simulink model "firefliesDemo"  (Simulink 7.4)
settings: Solver=ode3  StartTime=0.0  StopTime=200  FixedStep=1  RelTol=1e-3
values from neighbouring files (symbols this model uses):
  K = 2.5    [firefliesDemo.mat]
  N = 5    [clusterDemo.mat]    (also in firefliesDemo.mat = 10)
  omega = 0.628318530718    [firefliesDemo.mat]
  rho0 = 10    [firefliesDemo.mat]
  threshold = 0.8    [firefliesDemo.mat]
  var = 0    [clusterDemo.mat]    (also in firefliesDemo.mat = 3)
(part 1 of 2)
settings Model: Creator=chepeadan  LastModifiedBy=chepeadan

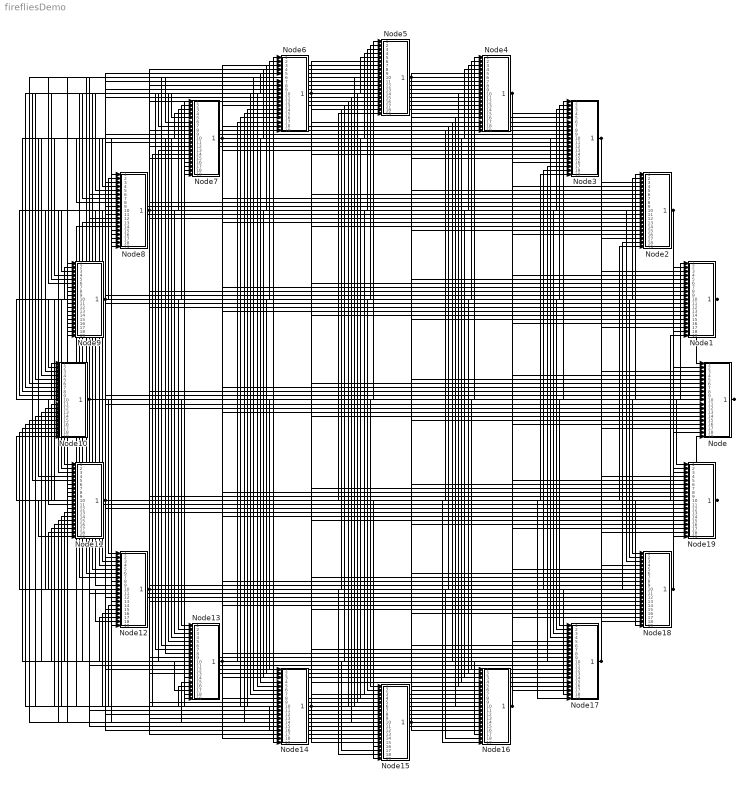
== system firefliesDemo ==
  Node : Subsystem
  Node1 : Subsystem
  Node10 : Subsystem
  Node11 : Subsystem
  Node12 : Subsystem
  Node13 : Subsystem
  Node14 : Subsystem
  Node15 : Subsystem
  Node16 : Subsystem
  Node17 : Subsystem
  Node18 : Subsystem
  Node19 : Subsystem
  Node2 : Subsystem
  Node3 : Subsystem
  Node4 : Subsystem
  Node5 : Subsystem
  Node6 : Subsystem
  Node7 : Subsystem
  Node8 : Subsystem
  Node9 : Subsystem
  wires:
  Node/1(Out1) -> Node1/1(In1), Node2/1(In1), Node3/1(In1), Node4/1(In1), Node5/1(In1), Node6/1(In1), Node7/1(In1), Node8/1(In1), Node9/1(In1), Node10/1(In1), Node11/1(In1), Node12/1(In1), Node13/1(In1), Node14/1(In1), Node15/1(In1), Node16/1(In1), Node17/1(In1), Node18/1(In1), Node19/1(In1)
  Node1/1(Out1) -> Node/1(In2), Node2/2(In2), Node3/2(In2), Node4/2(In2), Node5/2(In2), Node6/2(In2), Node7/2(In2), Node8/2(In2), Node9/2(In2), Node10/2(In2), Node11/2(In2), Node12/2(In2), Node13/2(In2), Node14/2(In2), Node15/2(In2), Node16/2(In2), Node17/2(In2), Node18/2(In2), Node19/2(In2)
  Node2/1(Out1) -> Node/2(In3), Node1/2(In3), Node3/3(In3), Node4/3(In3), Node5/3(In3), Node6/3(In3), Node7/3(In3), Node8/3(In3), Node9/3(In3), Node10/3(In3), Node11/3(In3), Node12/3(In3), Node13/3(In3), Node14/3(In3), Node15/3(In3), Node16/3(In3), Node17/3(In3), Node18/3(In3), Node19/3(In3)
  Node3/1(Out1) -> Node/3(In4), Node1/3(In4), Node2/3(In4), Node4/4(In4), Node5/4(In4), Node6/4(In4), Node7/4(In4), Node8/4(In4), Node9/4(In4), Node10/4(In4), Node11/4(In4), Node12/4(In4), Node13/4(In4), Node14/4(In4), Node15/4(In4), Node16/4(In4), Node17/4(In4), Node18/4(In4), Node19/4(In4)
  Node4/1(Out1) -> Node/4(In5), Node1/4(In5), Node2/4(In5), Node3/4(In5), Node5/5(In5), Node6/5(In5), Node7/5(In5), Node8/5(In5), Node9/5(In5), Node10/5(In5), Node11/5(In5), Node12/5(In5), Node13/5(In5), Node14/5(In5), Node15/5(In5), Node16/5(In5), Node17/5(In5), Node18/5(In5), Node19/5(In5)
  Node5/1(Out1) -> Node/5(In6), Node1/5(In6), Node2/5(In6), Node3/5(In6), Node4/5(In6), Node6/6(In6), Node7/6(In6), Node8/6(In6), Node9/6(In6), Node10/6(In6), Node11/6(In6), Node12/6(In6), Node13/6(In6), Node14/6(In6), Node15/6(In6), Node16/6(In6), Node17/6(In6), Node18/6(In6), Node19/6(In6)
  Node6/1(Out1) -> Node/6(In7), Node1/6(In7), Node2/6(In7), Node3/6(In7), Node4/6(In7), Node5/6(In7), Node7/7(In7), Node8/7(In7), Node9/7(In7), Node10/7(In7), Node11/7(In7), Node12/7(In7), Node13/7(In7), Node14/7(In7), Node15/7(In7), Node16/7(In7), Node17/7(In7), Node18/7(In7), Node19/7(In7)
  Node7/1(Out1) -> Node/7(In8), Node1/7(In8), Node2/7(In8), Node3/7(In8), Node4/7(In8), Node5/7(In8), Node6/7(In8), Node8/8(In8), Node9/8(In8), Node10/8(In8), Node11/8(In8), Node12/8(In8), Node13/8(In8), Node14/8(In8), Node15/8(In8), Node16/8(In8), Node17/8(In8), Node18/8(In8), Node19/8(In8)
  Node8/1(Out1) -> Node/8(In9), Node1/8(In9), Node2/8(In9), Node3/8(In9), Node4/8(In9), Node5/8(In9), Node6/8(In9), Node7/8(In9), Node9/9(In9), Node10/9(In9), Node11/9(In9), Node12/9(In9), Node13/9(In9), Node14/9(In9), Node15/9(In9), Node16/9(In9), Node17/9(In9), Node18/9(In9), Node19/9(In9)
  Node9/1(Out1) -> Node/9(In10), Node1/9(In10), Node2/9(In10), Node3/9(In10), Node4/9(In10), Node5/9(In10), Node6/9(In10), Node7/9(In10), Node8/9(In10), Node10/10(In10), Node11/10(In10), Node12/10(In10), Node13/10(In10), Node14/10(In10), Node15/10(In10), Node16/10(In10), Node17/10(In10), Node18/10(In10), Node19/10(In10)
  Node10/1(Out1) -> Node/10(In11), Node1/10(In11), Node2/10(In11), Node3/10(In11), Node4/10(In11), Node5/10(In11), Node6/10(In11), Node7/10(In11), Node8/10(In11), Node9/10(In11), Node11/11(In11), Node12/11(In11), Node13/11(In11), Node14/11(In11), Node15/11(In11), Node16/11(In11), Node17/11(In11), Node18/11(In11), Node19/11(In11)
  Node11/1(Out1) -> Node/11(In12), Node1/11(In12), Node2/11(In12), Node3/11(In12), Node4/11(In12), Node5/11(In12), Node6/11(In12), Node7/11(In12), Node8/11(In12), Node9/11(In12), Node10/11(In12), Node12/12(In12), Node13/12(In12), Node14/12(In12), Node15/12(In12), Node16/12(In12), Node17/12(In12), Node18/12(In12), Node19/12(In12)
  Node12/1(Out1) -> Node/12(In13), Node1/12(In13), Node2/12(In13), Node3/12(In13), Node4/12(In13), Node5/12(In13), Node6/12(In13), Node7/12(In13), Node8/12(In13), Node9/12(In13), Node10/12(In13), Node11/12(In13), Node13/13(In13), Node14/13(In13), Node15/13(In13), Node16/13(In13), Node17/13(In13), Node18/13(In13), Node19/13(In13)
  Node13/1(Out1) -> Node/13(In14), Node1/13(In14), Node2/13(In14), Node3/13(In14), Node4/13(In14), Node5/13(In14), Node6/13(In14), Node7/13(In14), Node8/13(In14), Node9/13(In14), Node10/13(In14), Node11/13(In14), Node12/13(In14), Node14/14(In14), Node15/14(In14), Node16/14(In14), Node17/14(In14), Node18/14(In14), Node19/14(In14)
  Node14/1(Out1) -> Node/14(In15), Node1/14(In15), Node2/14(In15), Node3/14(In15), Node4/14(In15), Node5/14(In15), Node6/14(In15), Node7/14(In15), Node8/14(In15), Node9/14(In15), Node10/14(In15), Node11/14(In15), Node12/14(In15), Node13/14(In15), Node15/15(In15), Node16/15(In15), Node17/15(In15), Node18/15(In15), Node19/15(In15)
  Node15/1(Out1) -> Node/15(In16), Node1/15(In16), Node2/15(In16), Node3/15(In16), Node4/15(In16), Node5/15(In16), Node6/15(In16), Node7/15(In16), Node8/15(In16), Node9/15(In16), Node10/15(In16), Node11/15(In16), Node12/15(In16), Node13/15(In16), Node14/15(In16), Node16/16(In16), Node17/16(In16), Node18/16(In16), Node19/16(In16)
  Node16/1(Out1) -> Node/16(In17), Node1/16(In17), Node2/16(In17), Node3/16(In17), Node4/16(In17), Node5/16(In17), Node6/16(In17), Node7/16(In17), Node8/16(In17), Node9/16(In17), Node10/16(In17), Node11/16(In17), Node12/16(In17), Node13/16(In17), Node14/16(In17), Node15/16(In17), Node17/17(In17), Node18/17(In17), Node19/17(In17)
  Node17/1(Out1) -> Node/17(In18), Node1/17(In18), Node2/17(In18), Node3/17(In18), Node4/17(In18), Node5/17(In18), Node6/17(In18), Node7/17(In18), Node8/17(In18), Node9/17(In18), Node10/17(In18), Node11/17(In18), Node12/17(In18), Node13/17(In18), Node14/17(In18), Node15/17(In18), Node16/17(In18), Node18/18(In18), Node19/18(In18)
  Node18/1(Out1) -> Node/18(In19), Node1/18(In19), Node2/18(In19), Node3/18(In19), Node4/18(In19), Node5/18(In19), Node6/18(In19), Node7/18(In19), Node8/18(In19), Node9/18(In19), Node10/18(In19), Node11/18(In19), Node12/18(In19), Node13/18(In19), Node14/18(In19), Node15/18(In19), Node16/18(In19), Node17/18(In19), Node19/19(In19)
  Node19/1(Out1) -> Node/19(In20), Node1/19(In20), Node2/19(In20), Node3/19(In20), Node4/19(In20), Node5/19(In20), Node6/19(In20), Node7/19(In20), Node8/19(In20), Node9/19(In20), Node10/19(In20), Node11/19(In20), Node12/19(In20), Node13/19(In20), Node14/19(In20), Node15/19(In20), Node16/19(In20), Node17/19(In20), Node18/19(In20)

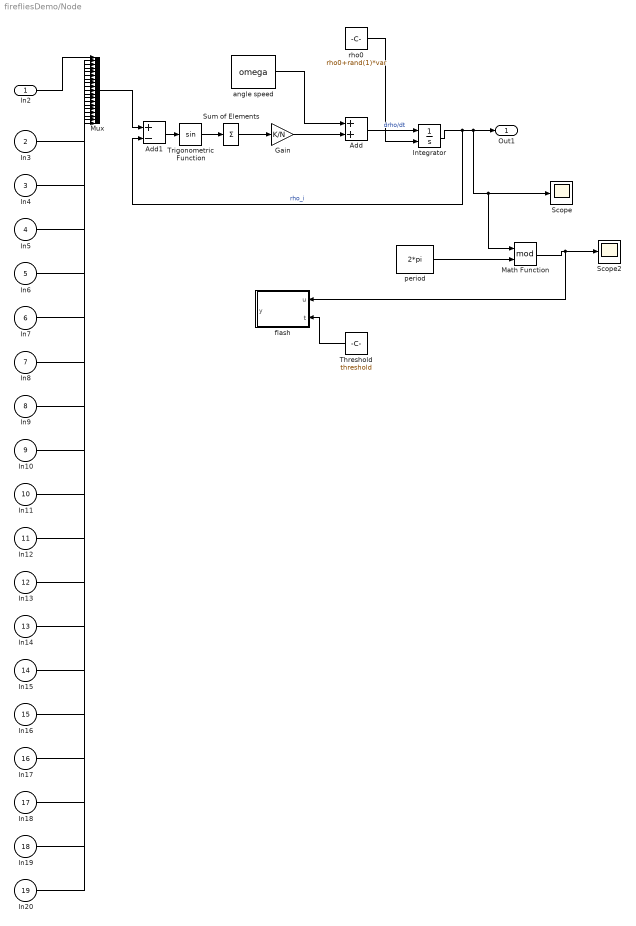
== system firefliesDemo/Node ==
  In2 : Inport  OutDataType=fixdt(1, 16)  OutScaling=2^0
  In3 : Inport  Port=2
  In4 : Inport  Port=3
  In5 : Inport  Port=4
  In6 : Inport  Port=5
  In7 : Inport  Port=6
  In8 : Inport  Port=7
  In9 : Inport  Port=8
  In10 : Inport  Port=9
  In11 : Inport  Port=10
  In12 : Inport  Port=11
  In13 : Inport  Port=12
  In14 : Inport  Port=13
  In15 : Inport  Port=14
  In16 : Inport  Port=15
  In17 : Inport  Port=16
  In18 : Inport  Port=17
  In19 : Inport  Port=18
  In20 : Inport  Port=19
  Add : Sum  OutDataType=fixdt(1, 16)  OutScaling=2^-10
  Add1 : Sum  Inputs=+-  OutDataType=fixdt(1, 16)  OutScaling=2^-10
  Gain : Gain  Gain=K/N  ParameterDataType=fixdt(1, 16)  ParameterScaling=2^0  OutDataType=fixdt(1, 16)  OutScaling=2^0
  Integrator : Integrator  InitialConditionSource=external
  Math Function : Math  Operator=mod  OutDataType=fixdt(1, 16)  OutScaling=2^0  SaturateOnIntegerOverflow=on
  Mux : Mux  Inputs=19
  Scope : Scope
  Scope2 : Scope
      settings: SaveName=ScopeData2
  Sum of Elements : Sum  Inputs=+  OutDataType=fixdt(1, 16)  OutScaling=2^-10
  Threshold : Constant  Value=threshold  OutDataType=fixdt(1, 16)  OutScaling=2^0
  Trigonometric Function : Trigonometry
  angle speed : Constant  Value=omega  OutDataType=fixdt(1, 16)  OutScaling=2^0
  flash : Stateflow chart
  period : Constant  Value=2*pi  OutDataType=fixdt(1, 16)  OutScaling=2^0
  rho0 : Constant  Value=rho0+rand(1)*var  OutDataType=fixdt(1, 16)  OutScaling=2^0
  Out1 : Outport  OutDataType=fixdt(1, 16)  OutScaling=2^0
  wires:
  In20/1 -> Mux/19
  In19/1 -> Mux/18
  In18/1 -> Mux/17
  In17/1 -> Mux/16
  In16/1 -> Mux/15
  In15/1 -> Mux/14
  In14/1 -> Mux/13
  In13/1 -> Mux/12
  In12/1 -> Mux/11
  In11/1 -> Mux/10
  In10/1 -> Mux/9
  In9/1 -> Mux/8
  In8/1 -> Mux/7
  In7/1 -> Mux/6
  In6/1 -> Mux/5
  In5/1 -> Mux/4
  In4/1 -> Mux/3
  In3/1 -> Mux/2
  Threshold/1 -> flash/2(t)
  Math Function/1 -> flash/1(u), Scope2/1
  period/1 -> Math Function/2
  rho0/1 -> Integrator/2
  Sum of Elements/1 -> Gain/1
  Trigonometric Function/1 -> Sum of Elements/1
  Add/1 -> Integrator/1  "drho/dt"
  Gain/1 -> Add/2
  angle speed/1 -> Add/1
  Add1/1 -> Trigonometric Function/1
  Integrator/1 -> Math Function/1, Scope/1, Out1/1, Add1/2  "rho_i"
  Mux/1 -> Add1/1
  In2/1 -> Mux/1

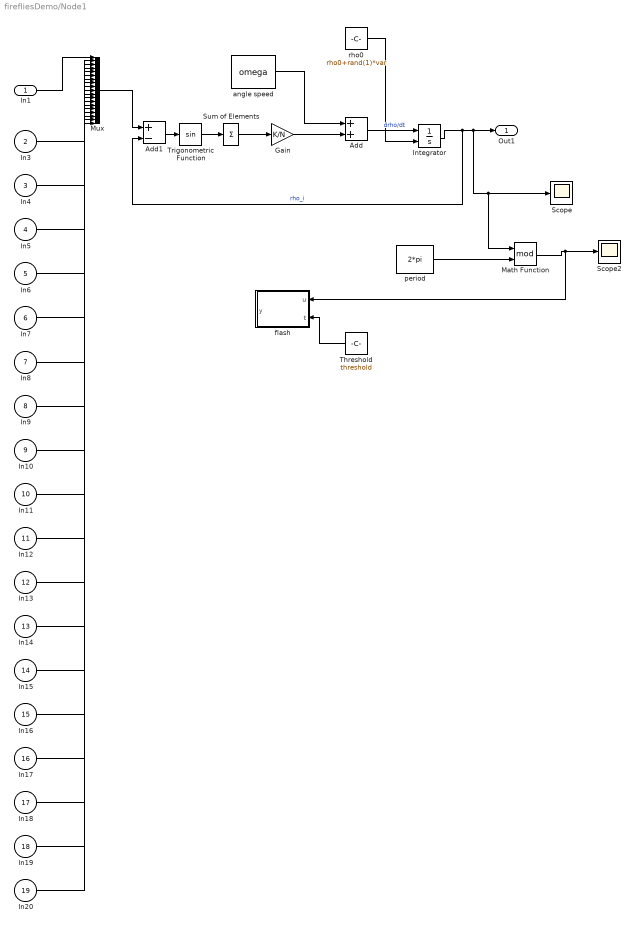
== system firefliesDemo/Node1 ==
  In1 : Inport  OutDataType=fixdt(1, 16)  OutScaling=2^0
  In3 : Inport  Port=2
  In4 : Inport  Port=3
  In5 : Inport  Port=4
  In6 : Inport  Port=5
  In7 : Inport  Port=6
  In8 : Inport  Port=7
  In9 : Inport  Port=8
  In10 : Inport  Port=9
  In11 : Inport  Port=10
  In12 : Inport  Port=11
  In13 : Inport  Port=12
  In14 : Inport  Port=13
  In15 : Inport  Port=14
  In16 : Inport  Port=15
  In17 : Inport  Port=16
  In18 : Inport  Port=17
  In19 : Inport  Port=18
  In20 : Inport  Port=19
  Add : Sum  OutDataType=fixdt(1, 16)  OutScaling=2^-10
  Add1 : Sum  Inputs=+-  OutDataType=fixdt(1, 16)  OutScaling=2^-10
  Gain : Gain  Gain=K/N  ParameterDataType=fixdt(1, 16)  ParameterScaling=2^0  OutDataType=fixdt(1, 16)  OutScaling=2^0
  Integrator : Integrator  InitialConditionSource=external
  Math Function : Math  Operator=mod  OutDataType=fixdt(1, 16)  OutScaling=2^0  SaturateOnIntegerOverflow=on
  Mux : Mux  Inputs=19
  Scope : Scope
  Scope2 : Scope
      settings: SaveName=ScopeData2
  Sum of Elements : Sum  Inputs=+  OutDataType=fixdt(1, 16)  OutScaling=2^-10
  Threshold : Constant  Value=threshold  OutDataType=fixdt(1, 16)  OutScaling=2^0
  Trigonometric Function : Trigonometry
  angle speed : Constant  Value=omega  OutDataType=fixdt(1, 16)  OutScaling=2^0
  flash : Stateflow chart
  period : Constant  Value=2*pi  OutDataType=fixdt(1, 16)  OutScaling=2^0
  rho0 : Constant  Value=rho0+rand(1)*var  OutDataType=fixdt(1, 16)  OutScaling=2^0
  Out1 : Outport  OutDataType=fixdt(1, 16)  OutScaling=2^0
  wires:
  In20/1 -> Mux/19
  In19/1 -> Mux/18
  In18/1 -> Mux/17
  In17/1 -> Mux/16
  In16/1 -> Mux/15
  In15/1 -> Mux/14
  In14/1 -> Mux/13
  In13/1 -> Mux/12
  In12/1 -> Mux/11
  In11/1 -> Mux/10
  In10/1 -> Mux/9
  In9/1 -> Mux/8
  In8/1 -> Mux/7
  In7/1 -> Mux/6
  In6/1 -> Mux/5
  In5/1 -> Mux/4
  In4/1 -> Mux/3
  In3/1 -> Mux/2
  Threshold/1 -> flash/2(t)
  Math Function/1 -> flash/1(u), Scope2/1
  period/1 -> Math Function/2
  rho0/1 -> Integrator/2
  Sum of Elements/1 -> Gain/1
  Trigonometric Function/1 -> Sum of Elements/1
  Add/1 -> Integrator/1  "drho/dt"
  Gain/1 -> Add/2
  angle speed/1 -> Add/1
  Add1/1 -> Trigonometric Function/1
  Integrator/1 -> Math Function/1, Scope/1, Out1/1, Add1/2  "rho_i"
  Mux/1 -> Add1/1
  In1/1 -> Mux/1

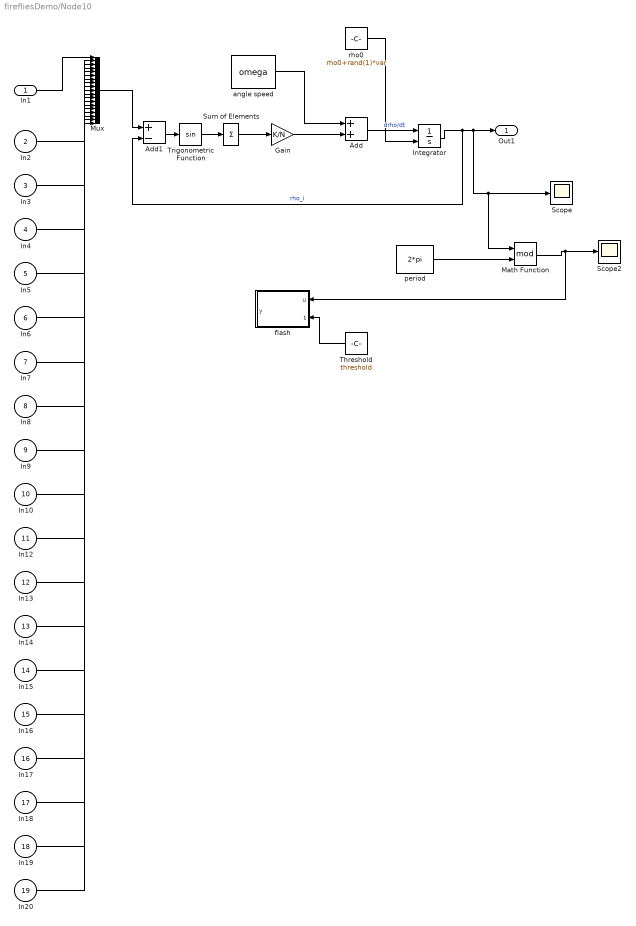
== system firefliesDemo/Node10 ==
  In1 : Inport  OutDataType=fixdt(1, 16)  OutScaling=2^0
  In2 : Inport  Port=2
  In3 : Inport  Port=3
  In4 : Inport  Port=4
  In5 : Inport  Port=5
  In6 : Inport  Port=6
  In7 : Inport  Port=7
  In8 : Inport  Port=8
  In9 : Inport  Port=9
  In10 : Inport  Port=10
  In12 : Inport  Port=11
  In13 : Inport  Port=12
  In14 : Inport  Port=13
  In15 : Inport  Port=14
  In16 : Inport  Port=15
  In17 : Inport  Port=16
  In18 : Inport  Port=17
  In19 : Inport  Port=18
  In20 : Inport  Port=19
  Add : Sum  OutDataType=fixdt(1, 16)  OutScaling=2^-10
  Add1 : Sum  Inputs=+-  OutDataType=fixdt(1, 16)  OutScaling=2^-10
  Gain : Gain  Gain=K/N  ParameterDataType=fixdt(1, 16)  ParameterScaling=2^0  OutDataType=fixdt(1, 16)  OutScaling=2^0
  Integrator : Integrator  InitialConditionSource=external
  Math Function : Math  Operator=mod  OutDataType=fixdt(1, 16)  OutScaling=2^0  SaturateOnIntegerOverflow=on
  Mux : Mux  Inputs=19
  Scope : Scope
  Scope2 : Scope
      settings: SaveName=ScopeData2
  Sum of Elements : Sum  Inputs=+  OutDataType=fixdt(1, 16)  OutScaling=2^-10
  Threshold : Constant  Value=threshold  OutDataType=fixdt(1, 16)  OutScaling=2^0
  Trigonometric Function : Trigonometry
  angle speed : Constant  Value=omega  OutDataType=fixdt(1, 16)  OutScaling=2^0
  flash : Stateflow chart
  period : Constant  Value=2*pi  OutDataType=fixdt(1, 16)  OutScaling=2^0
  rho0 : Constant  Value=rho0+rand(1)*var  OutDataType=fixdt(1, 16)  OutScaling=2^0
  Out1 : Outport  OutDataType=fixdt(1, 16)  OutScaling=2^0
  wires:
  In20/1 -> Mux/19
  In19/1 -> Mux/18
  In18/1 -> Mux/17
  In17/1 -> Mux/16
  In16/1 -> Mux/15
  In15/1 -> Mux/14
  In14/1 -> Mux/13
  In13/1 -> Mux/12
  In12/1 -> Mux/11
  In10/1 -> Mux/10
  In9/1 -> Mux/9
  In8/1 -> Mux/8
  In7/1 -> Mux/7
  In6/1 -> Mux/6
  In5/1 -> Mux/5
  In4/1 -> Mux/4
  In3/1 -> Mux/3
  In2/1 -> Mux/2
  Threshold/1 -> flash/2(t)
  Math Function/1 -> flash/1(u), Scope2/1
  period/1 -> Math Function/2
  rho0/1 -> Integrator/2
  Sum of Elements/1 -> Gain/1
  Trigonometric Function/1 -> Sum of Elements/1
  Add/1 -> Integrator/1  "drho/dt"
  Gain/1 -> Add/2
  angle speed/1 -> Add/1
  Add1/1 -> Trigonometric Function/1
  Integrator/1 -> Math Function/1, Scope/1, Out1/1, Add1/2  "rho_i"
  Mux/1 -> Add1/1
  In1/1 -> Mux/1

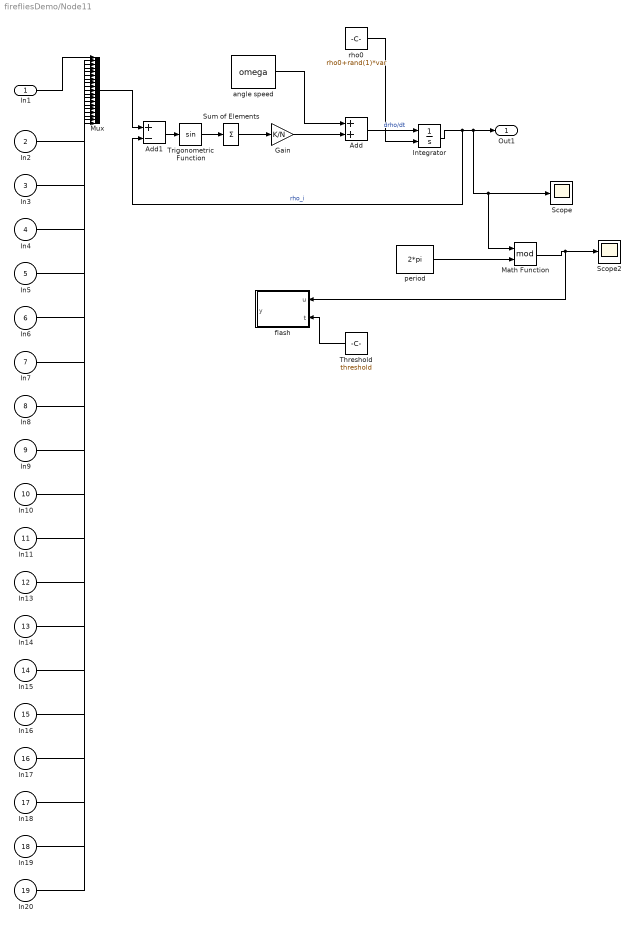
== system firefliesDemo/Node11 ==
  In1 : Inport  OutDataType=fixdt(1, 16)  OutScaling=2^0
  In2 : Inport  Port=2
  In3 : Inport  Port=3
  In4 : Inport  Port=4
  In5 : Inport  Port=5
  In6 : Inport  Port=6
  In7 : Inport  Port=7
  In8 : Inport  Port=8
  In9 : Inport  Port=9
  In10 : Inport  Port=10
  In11 : Inport  Port=11
  In13 : Inport  Port=12
  In14 : Inport  Port=13
  In15 : Inport  Port=14
  In16 : Inport  Port=15
  In17 : Inport  Port=16
  In18 : Inport  Port=17
  In19 : Inport  Port=18
  In20 : Inport  Port=19
  Add : Sum  OutDataType=fixdt(1, 16)  OutScaling=2^-10
  Add1 : Sum  Inputs=+-  OutDataType=fixdt(1, 16)  OutScaling=2^-10
  Gain : Gain  Gain=K/N  ParameterDataType=fixdt(1, 16)  ParameterScaling=2^0  OutDataType=fixdt(1, 16)  OutScaling=2^0
  Integrator : Integrator  InitialConditionSource=external
  Math Function : Math  Operator=mod  OutDataType=fixdt(1, 16)  OutScaling=2^0  SaturateOnIntegerOverflow=on
  Mux : Mux  Inputs=19
  Scope : Scope
  Scope2 : Scope
      settings: SaveName=ScopeData2
  Sum of Elements : Sum  Inputs=+  OutDataType=fixdt(1, 16)  OutScaling=2^-10
  Threshold : Constant  Value=threshold  OutDataType=fixdt(1, 16)  OutScaling=2^0
  Trigonometric Function : Trigonometry
  angle speed : Constant  Value=omega  OutDataType=fixdt(1, 16)  OutScaling=2^0
  flash : Stateflow chart
  period : Constant  Value=2*pi  OutDataType=fixdt(1, 16)  OutScaling=2^0
  rho0 : Constant  Value=rho0+rand(1)*var  OutDataType=fixdt(1, 16)  OutScaling=2^0
  Out1 : Outport  OutDataType=fixdt(1, 16)  OutScaling=2^0
  wires:
  In20/1 -> Mux/19
  In19/1 -> Mux/18
  In18/1 -> Mux/17
  In17/1 -> Mux/16
  In16/1 -> Mux/15
  In15/1 -> Mux/14
  In14/1 -> Mux/13
  In13/1 -> Mux/12
  In11/1 -> Mux/11
  In10/1 -> Mux/10
  In9/1 -> Mux/9
  In8/1 -> Mux/8
  In7/1 -> Mux/7
  In6/1 -> Mux/6
  In5/1 -> Mux/5
  In4/1 -> Mux/4
  In3/1 -> Mux/3
  In2/1 -> Mux/2
  Threshold/1 -> flash/2(t)
  Math Function/1 -> flash/1(u), Scope2/1
  period/1 -> Math Function/2
  rho0/1 -> Integrator/2
  Sum of Elements/1 -> Gain/1
  Trigonometric Function/1 -> Sum of Elements/1
  Add/1 -> Integrator/1  "drho/dt"
  Gain/1 -> Add/2
  angle speed/1 -> Add/1
  Add1/1 -> Trigonometric Function/1
  Integrator/1 -> Math Function/1, Scope/1, Out1/1, Add1/2  "rho_i"
  Mux/1 -> Add1/1
  In1/1 -> Mux/1

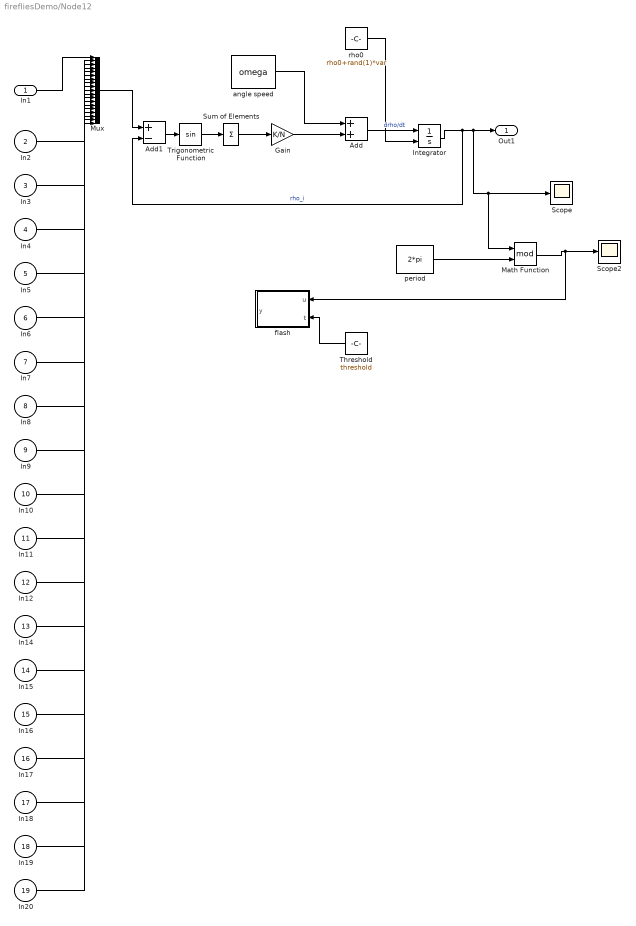
== system firefliesDemo/Node12 ==
  In1 : Inport  OutDataType=fixdt(1, 16)  OutScaling=2^0
  In2 : Inport  Port=2
  In3 : Inport  Port=3
  In4 : Inport  Port=4
  In5 : Inport  Port=5
  In6 : Inport  Port=6
  In7 : Inport  Port=7
  In8 : Inport  Port=8
  In9 : Inport  Port=9
  In10 : Inport  Port=10
  In11 : Inport  Port=11
  In12 : Inport  Port=12
  In14 : Inport  Port=13
  In15 : Inport  Port=14
  In16 : Inport  Port=15
  In17 : Inport  Port=16
  In18 : Inport  Port=17
  In19 : Inport  Port=18
  In20 : Inport  Port=19
  Add : Sum  OutDataType=fixdt(1, 16)  OutScaling=2^-10
  Add1 : Sum  Inputs=+-  OutDataType=fixdt(1, 16)  OutScaling=2^-10
  Gain : Gain  Gain=K/N  ParameterDataType=fixdt(1, 16)  ParameterScaling=2^0  OutDataType=fixdt(1, 16)  OutScaling=2^0
  Integrator : Integrator  InitialConditionSource=external
  Math Function : Math  Operator=mod  OutDataType=fixdt(1, 16)  OutScaling=2^0  SaturateOnIntegerOverflow=on
  Mux : Mux  Inputs=19
  Scope : Scope
  Scope2 : Scope
      settings: SaveName=ScopeData2
  Sum of Elements : Sum  Inputs=+  OutDataType=fixdt(1, 16)  OutScaling=2^-10
  Threshold : Constant  Value=threshold  OutDataType=fixdt(1, 16)  OutScaling=2^0
  Trigonometric Function : Trigonometry
  angle speed : Constant  Value=omega  OutDataType=fixdt(1, 16)  OutScaling=2^0
  flash : Stateflow chart
  period : Constant  Value=2*pi  OutDataType=fixdt(1, 16)  OutScaling=2^0
  rho0 : Constant  Value=rho0+rand(1)*var  OutDataType=fixdt(1, 16)  OutScaling=2^0
  Out1 : Outport  OutDataType=fixdt(1, 16)  OutScaling=2^0
  wires:
  In20/1 -> Mux/19
  In19/1 -> Mux/18
  In18/1 -> Mux/17
  In17/1 -> Mux/16
  In16/1 -> Mux/15
  In15/1 -> Mux/14
  In14/1 -> Mux/13
  In12/1 -> Mux/12
  In11/1 -> Mux/11
  In10/1 -> Mux/10
  In9/1 -> Mux/9
  In8/1 -> Mux/8
  In7/1 -> Mux/7
  In6/1 -> Mux/6
  In5/1 -> Mux/5
  In4/1 -> Mux/4
  In3/1 -> Mux/3
  In2/1 -> Mux/2
  Threshold/1 -> flash/2(t)
  Math Function/1 -> flash/1(u), Scope2/1
  period/1 -> Math Function/2
  rho0/1 -> Integrator/2
  Sum of Elements/1 -> Gain/1
  Trigonometric Function/1 -> Sum of Elements/1
  Add/1 -> Integrator/1  "drho/dt"
  Gain/1 -> Add/2
  angle speed/1 -> Add/1
  Add1/1 -> Trigonometric Function/1
  Integrator/1 -> Math Function/1, Scope/1, Out1/1, Add1/2  "rho_i"
  Mux/1 -> Add1/1
  In1/1 -> Mux/1

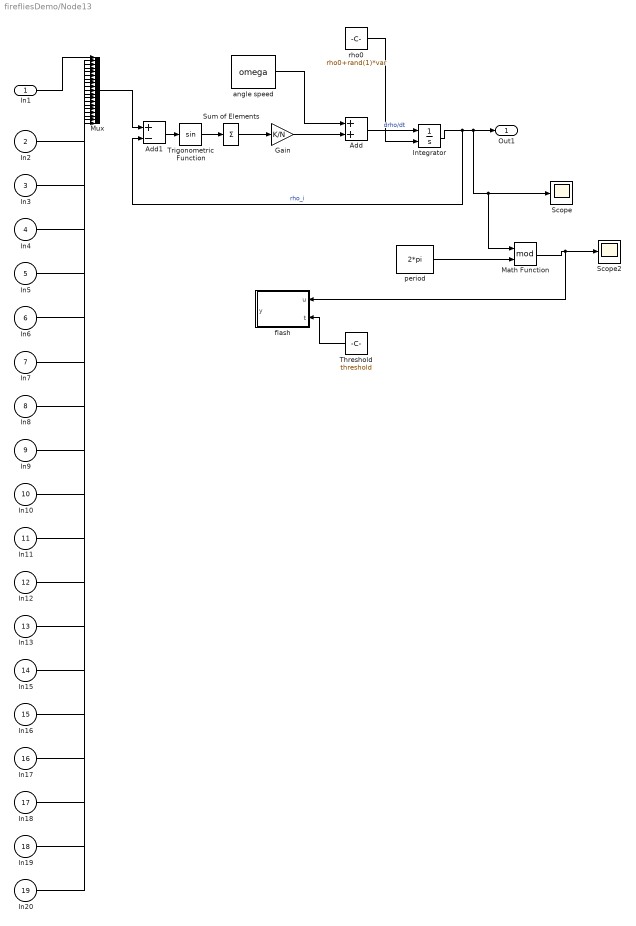
== system firefliesDemo/Node13 ==
  In1 : Inport  OutDataType=fixdt(1, 16)  OutScaling=2^0
  In2 : Inport  Port=2
  In3 : Inport  Port=3
  In4 : Inport  Port=4
  In5 : Inport  Port=5
  In6 : Inport  Port=6
  In7 : Inport  Port=7
  In8 : Inport  Port=8
  In9 : Inport  Port=9
  In10 : Inport  Port=10
  In11 : Inport  Port=11
  In12 : Inport  Port=12
  In13 : Inport  Port=13
  In15 : Inport  Port=14
  In16 : Inport  Port=15
  In17 : Inport  Port=16
  In18 : Inport  Port=17
  In19 : Inport  Port=18
  In20 : Inport  Port=19
  Add : Sum  OutDataType=fixdt(1, 16)  OutScaling=2^-10
  Add1 : Sum  Inputs=+-  OutDataType=fixdt(1, 16)  OutScaling=2^-10
  Gain : Gain  Gain=K/N  ParameterDataType=fixdt(1, 16)  ParameterScaling=2^0  OutDataType=fixdt(1, 16)  OutScaling=2^0
  Integrator : Integrator  InitialConditionSource=external
  Math Function : Math  Operator=mod  OutDataType=fixdt(1, 16)  OutScaling=2^0  SaturateOnIntegerOverflow=on
  Mux : Mux  Inputs=19
  Scope : Scope
  Scope2 : Scope
      settings: SaveName=ScopeData2
  Sum of Elements : Sum  Inputs=+  OutDataType=fixdt(1, 16)  OutScaling=2^-10
  Threshold : Constant  Value=threshold  OutDataType=fixdt(1, 16)  OutScaling=2^0
  Trigonometric Function : Trigonometry
  angle speed : Constant  Value=omega  OutDataType=fixdt(1, 16)  OutScaling=2^0
  flash : Stateflow chart
  period : Constant  Value=2*pi  OutDataType=fixdt(1, 16)  OutScaling=2^0
  rho0 : Constant  Value=rho0+rand(1)*var  OutDataType=fixdt(1, 16)  OutScaling=2^0
  Out1 : Outport  OutDataType=fixdt(1, 16)  OutScaling=2^0
  wires:
  In20/1 -> Mux/19
  In19/1 -> Mux/18
  In18/1 -> Mux/17
  In17/1 -> Mux/16
  In16/1 -> Mux/15
  In15/1 -> Mux/14
  In13/1 -> Mux/13
  In12/1 -> Mux/12
  In11/1 -> Mux/11
  In10/1 -> Mux/10
  In9/1 -> Mux/9
  In8/1 -> Mux/8
  In7/1 -> Mux/7
  In6/1 -> Mux/6
  In5/1 -> Mux/5
  In4/1 -> Mux/4
  In3/1 -> Mux/3
  In2/1 -> Mux/2
  Threshold/1 -> flash/2(t)
  Math Function/1 -> flash/1(u), Scope2/1
  period/1 -> Math Function/2
  rho0/1 -> Integrator/2
  Sum of Elements/1 -> Gain/1
  Trigonometric Function/1 -> Sum of Elements/1
  Add/1 -> Integrator/1  "drho/dt"
  Gain/1 -> Add/2
  angle speed/1 -> Add/1
  Add1/1 -> Trigonometric Function/1
  Integrator/1 -> Math Function/1, Scope/1, Out1/1, Add1/2  "rho_i"
  Mux/1 -> Add1/1
  In1/1 -> Mux/1

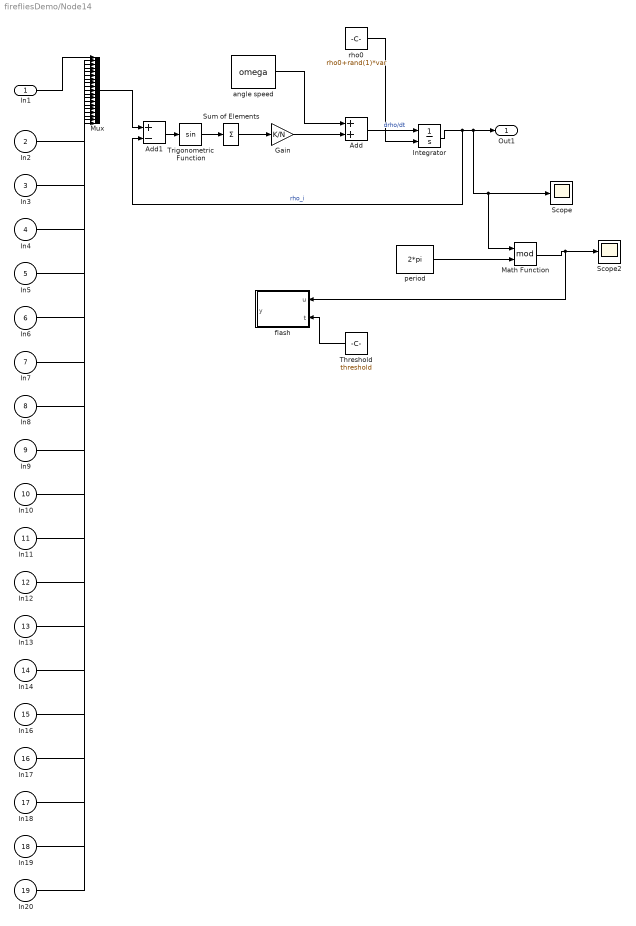
== system firefliesDemo/Node14 ==
  In1 : Inport  OutDataType=fixdt(1, 16)  OutScaling=2^0
  In2 : Inport  Port=2
  In3 : Inport  Port=3
  In4 : Inport  Port=4
  In5 : Inport  Port=5
  In6 : Inport  Port=6
  In7 : Inport  Port=7
  In8 : Inport  Port=8
  In9 : Inport  Port=9
  In10 : Inport  Port=10
  In11 : Inport  Port=11
  In12 : Inport  Port=12
  In13 : Inport  Port=13
  In14 : Inport  Port=14
  In16 : Inport  Port=15
  In17 : Inport  Port=16
  In18 : Inport  Port=17
  In19 : Inport  Port=18
  In20 : Inport  Port=19
  Add : Sum  OutDataType=fixdt(1, 16)  OutScaling=2^-10
  Add1 : Sum  Inputs=+-  OutDataType=fixdt(1, 16)  OutScaling=2^-10
  Gain : Gain  Gain=K/N  ParameterDataType=fixdt(1, 16)  ParameterScaling=2^0  OutDataType=fixdt(1, 16)  OutScaling=2^0
  Integrator : Integrator  InitialConditionSource=external
  Math Function : Math  Operator=mod  OutDataType=fixdt(1, 16)  OutScaling=2^0  SaturateOnIntegerOverflow=on
  Mux : Mux  Inputs=19
  Scope : Scope
  Scope2 : Scope
      settings: SaveName=ScopeData2
  Sum of Elements : Sum  Inputs=+  OutDataType=fixdt(1, 16)  OutScaling=2^-10
  Threshold : Constant  Value=threshold  OutDataType=fixdt(1, 16)  OutScaling=2^0
  Trigonometric Function : Trigonometry
  angle speed : Constant  Value=omega  OutDataType=fixdt(1, 16)  OutScaling=2^0
  flash : Stateflow chart
  period : Constant  Value=2*pi  OutDataType=fixdt(1, 16)  OutScaling=2^0
  rho0 : Constant  Value=rho0+rand(1)*var  OutDataType=fixdt(1, 16)  OutScaling=2^0
  Out1 : Outport  OutDataType=fixdt(1, 16)  OutScaling=2^0
  wires:
  In20/1 -> Mux/19
  In19/1 -> Mux/18
  In18/1 -> Mux/17
  In17/1 -> Mux/16
  In16/1 -> Mux/15
  In14/1 -> Mux/14
  In13/1 -> Mux/13
  In12/1 -> Mux/12
  In11/1 -> Mux/11
  In10/1 -> Mux/10
  In9/1 -> Mux/9
  In8/1 -> Mux/8
  In7/1 -> Mux/7
  In6/1 -> Mux/6
  In5/1 -> Mux/5
  In4/1 -> Mux/4
  In3/1 -> Mux/3
  In2/1 -> Mux/2
  Threshold/1 -> flash/2(t)
  Math Function/1 -> flash/1(u), Scope2/1
  period/1 -> Math Function/2
  rho0/1 -> Integrator/2
  Sum of Elements/1 -> Gain/1
  Trigonometric Function/1 -> Sum of Elements/1
  Add/1 -> Integrator/1  "drho/dt"
  Gain/1 -> Add/2
  angle speed/1 -> Add/1
  Add1/1 -> Trigonometric Function/1
  Integrator/1 -> Math Function/1, Scope/1, Out1/1, Add1/2  "rho_i"
  Mux/1 -> Add1/1
  In1/1 -> Mux/1

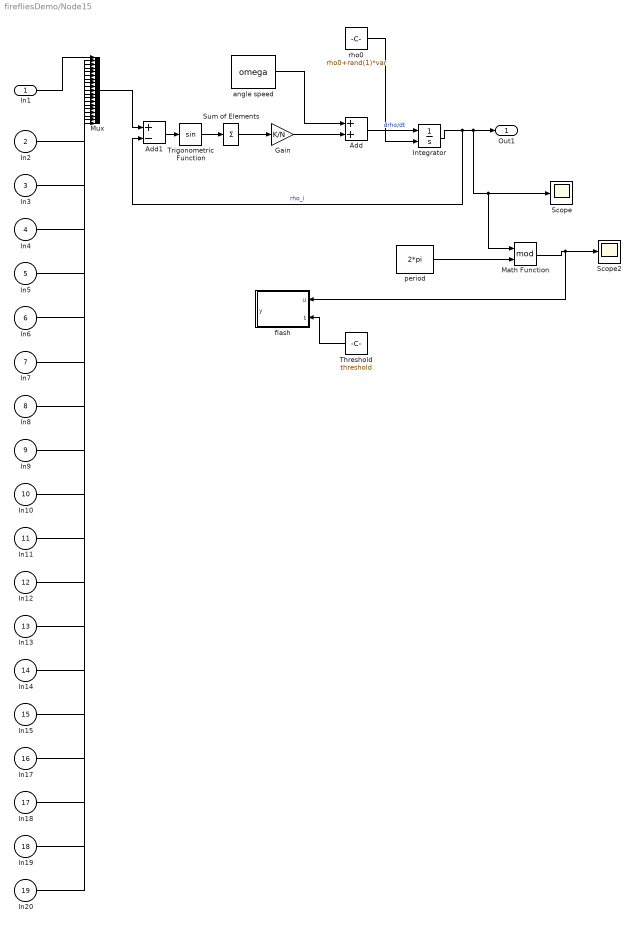
== system firefliesDemo/Node15 ==
  In1 : Inport  OutDataType=fixdt(1, 16)  OutScaling=2^0
  In2 : Inport  Port=2
  In3 : Inport  Port=3
  In4 : Inport  Port=4
  In5 : Inport  Port=5
  In6 : Inport  Port=6
  In7 : Inport  Port=7
  In8 : Inport  Port=8
  In9 : Inport  Port=9
  In10 : Inport  Port=10
  In11 : Inport  Port=11
  In12 : Inport  Port=12
  In13 : Inport  Port=13
  In14 : Inport  Port=14
  In15 : Inport  Port=15
  In17 : Inport  Port=16
  In18 : Inport  Port=17
  In19 : Inport  Port=18
  In20 : Inport  Port=19
  Add : Sum  OutDataType=fixdt(1, 16)  OutScaling=2^-10
  Add1 : Sum  Inputs=+-  OutDataType=fixdt(1, 16)  OutScaling=2^-10
  Gain : Gain  Gain=K/N  ParameterDataType=fixdt(1, 16)  ParameterScaling=2^0  OutDataType=fixdt(1, 16)  OutScaling=2^0
  Integrator : Integrator  InitialConditionSource=external
  Math Function : Math  Operator=mod  OutDataType=fixdt(1, 16)  OutScaling=2^0  SaturateOnIntegerOverflow=on
  Mux : Mux  Inputs=19
  Scope : Scope
  Scope2 : Scope
      settings: SaveName=ScopeData2
  Sum of Elements : Sum  Inputs=+  OutDataType=fixdt(1, 16)  OutScaling=2^-10
  Threshold : Constant  Value=threshold  OutDataType=fixdt(1, 16)  OutScaling=2^0
  Trigonometric Function : Trigonometry
  angle speed : Constant  Value=omega  OutDataType=fixdt(1, 16)  OutScaling=2^0
  flash : Stateflow chart
  period : Constant  Value=2*pi  OutDataType=fixdt(1, 16)  OutScaling=2^0
  rho0 : Constant  Value=rho0+rand(1)*var  OutDataType=fixdt(1, 16)  OutScaling=2^0
  Out1 : Outport  OutDataType=fixdt(1, 16)  OutScaling=2^0
  wires:
  In20/1 -> Mux/19
  In19/1 -> Mux/18
  In18/1 -> Mux/17
  In17/1 -> Mux/16
  In15/1 -> Mux/15
  In14/1 -> Mux/14
  In13/1 -> Mux/13
  In12/1 -> Mux/12
  In11/1 -> Mux/11
  In10/1 -> Mux/10
  In9/1 -> Mux/9
  In8/1 -> Mux/8
  In7/1 -> Mux/7
  In6/1 -> Mux/6
  In5/1 -> Mux/5
  In4/1 -> Mux/4
  In3/1 -> Mux/3
  In2/1 -> Mux/2
  Threshold/1 -> flash/2(t)
  Math Function/1 -> flash/1(u), Scope2/1
  period/1 -> Math Function/2
  rho0/1 -> Integrator/2
  Sum of Elements/1 -> Gain/1
  Trigonometric Function/1 -> Sum of Elements/1
  Add/1 -> Integrator/1  "drho/dt"
  Gain/1 -> Add/2
  angle speed/1 -> Add/1
  Add1/1 -> Trigonometric Function/1
  Integrator/1 -> Math Function/1, Scope/1, Out1/1, Add1/2  "rho_i"
  Mux/1 -> Add1/1
  In1/1 -> Mux/1

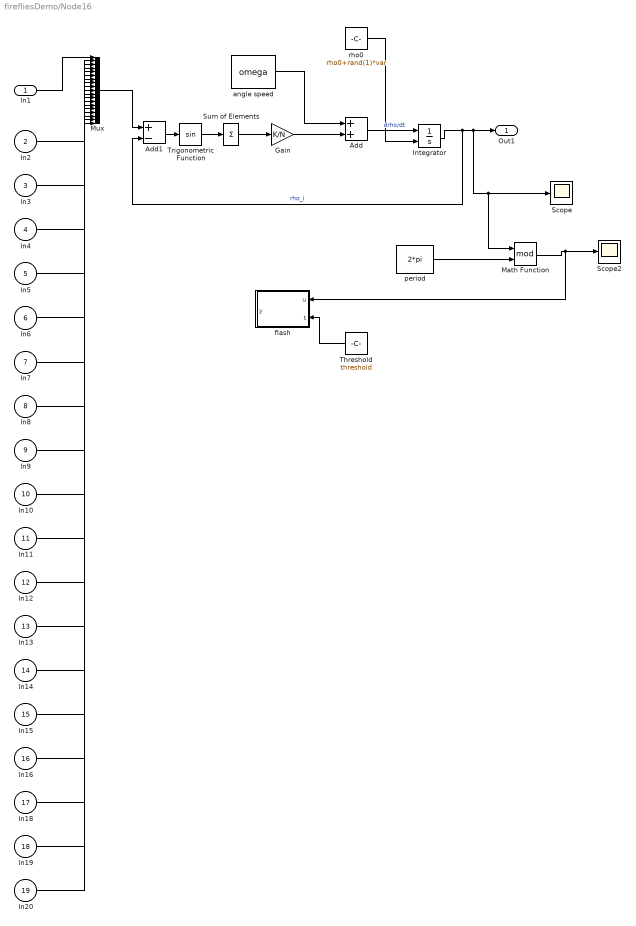
== system firefliesDemo/Node16 ==
  In1 : Inport  OutDataType=fixdt(1, 16)  OutScaling=2^0
  In2 : Inport  Port=2
  In3 : Inport  Port=3
  In4 : Inport  Port=4
  In5 : Inport  Port=5
  In6 : Inport  Port=6
  In7 : Inport  Port=7
  In8 : Inport  Port=8
  In9 : Inport  Port=9
  In10 : Inport  Port=10
  In11 : Inport  Port=11
  In12 : Inport  Port=12
  In13 : Inport  Port=13
  In14 : Inport  Port=14
  In15 : Inport  Port=15
  In16 : Inport  Port=16
  In18 : Inport  Port=17
  In19 : Inport  Port=18
  In20 : Inport  Port=19
  Add : Sum  OutDataType=fixdt(1, 16)  OutScaling=2^-10
  Add1 : Sum  Inputs=+-  OutDataType=fixdt(1, 16)  OutScaling=2^-10
  Gain : Gain  Gain=K/N  ParameterDataType=fixdt(1, 16)  ParameterScaling=2^0  OutDataType=fixdt(1, 16)  OutScaling=2^0
  Integrator : Integrator  InitialConditionSource=external
  Math Function : Math  Operator=mod  OutDataType=fixdt(1, 16)  OutScaling=2^0  SaturateOnIntegerOverflow=on
  Mux : Mux  Inputs=19
  Scope : Scope
  Scope2 : Scope
      settings: SaveName=ScopeData2
  Sum of Elements : Sum  Inputs=+  OutDataType=fixdt(1, 16)  OutScaling=2^-10
  Threshold : Constant  Value=threshold  OutDataType=fixdt(1, 16)  OutScaling=2^0
  Trigonometric Function : Trigonometry
  angle speed : Constant  Value=omega  OutDataType=fixdt(1, 16)  OutScaling=2^0
  flash : Stateflow chart
  period : Constant  Value=2*pi  OutDataType=fixdt(1, 16)  OutScaling=2^0
  rho0 : Constant  Value=rho0+rand(1)*var  OutDataType=fixdt(1, 16)  OutScaling=2^0
  Out1 : Outport  OutDataType=fixdt(1, 16)  OutScaling=2^0
  wires:
  In20/1 -> Mux/19
  In19/1 -> Mux/18
  In18/1 -> Mux/17
  In16/1 -> Mux/16
  In15/1 -> Mux/15
  In14/1 -> Mux/14
  In13/1 -> Mux/13
  In12/1 -> Mux/12
  In11/1 -> Mux/11
  In10/1 -> Mux/10
  In9/1 -> Mux/9
  In8/1 -> Mux/8
  In7/1 -> Mux/7
  In6/1 -> Mux/6
  In5/1 -> Mux/5
  In4/1 -> Mux/4
  In3/1 -> Mux/3
  In2/1 -> Mux/2
  Threshold/1 -> flash/2(t)
  Math Function/1 -> flash/1(u), Scope2/1
  period/1 -> Math Function/2
  rho0/1 -> Integrator/2
  Sum of Elements/1 -> Gain/1
  Trigonometric Function/1 -> Sum of Elements/1
  Add/1 -> Integrator/1  "drho/dt"
  Gain/1 -> Add/2
  angle speed/1 -> Add/1
  Add1/1 -> Trigonometric Function/1
  Integrator/1 -> Math Function/1, Scope/1, Out1/1, Add1/2  "rho_i"
  Mux/1 -> Add1/1
  In1/1 -> Mux/1

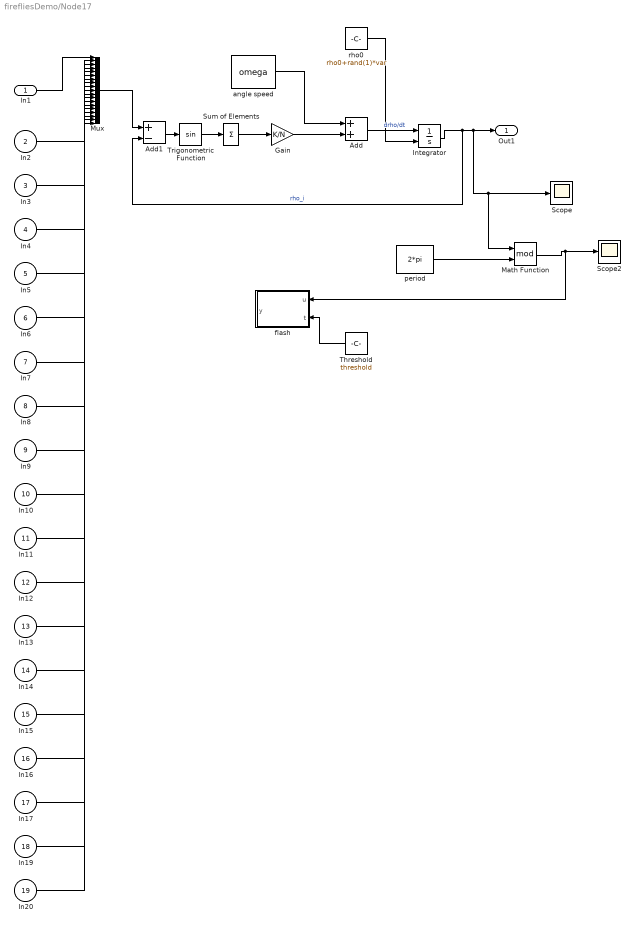
== system firefliesDemo/Node17 ==
  In1 : Inport  OutDataType=fixdt(1, 16)  OutScaling=2^0
  In2 : Inport  Port=2
  In3 : Inport  Port=3
  In4 : Inport  Port=4
  In5 : Inport  Port=5
  In6 : Inport  Port=6
  In7 : Inport  Port=7
  In8 : Inport  Port=8
  In9 : Inport  Port=9
  In10 : Inport  Port=10
  In11 : Inport  Port=11
  In12 : Inport  Port=12
  In13 : Inport  Port=13
  In14 : Inport  Port=14
  In15 : Inport  Port=15
  In16 : Inport  Port=16
  In17 : Inport  Port=17
  In19 : Inport  Port=18
  In20 : Inport  Port=19
  Add : Sum  OutDataType=fixdt(1, 16)  OutScaling=2^-10
  Add1 : Sum  Inputs=+-  OutDataType=fixdt(1, 16)  OutScaling=2^-10
  Gain : Gain  Gain=K/N  ParameterDataType=fixdt(1, 16)  ParameterScaling=2^0  OutDataType=fixdt(1, 16)  OutScaling=2^0
  Integrator : Integrator  InitialConditionSource=external
  Math Function : Math  Operator=mod  OutDataType=fixdt(1, 16)  OutScaling=2^0  SaturateOnIntegerOverflow=on
  Mux : Mux  Inputs=19
  Scope : Scope
  Scope2 : Scope
      settings: SaveName=ScopeData2
  Sum of Elements : Sum  Inputs=+  OutDataType=fixdt(1, 16)  OutScaling=2^-10
  Threshold : Constant  Value=threshold  OutDataType=fixdt(1, 16)  OutScaling=2^0
  Trigonometric Function : Trigonometry
  angle speed : Constant  Value=omega  OutDataType=fixdt(1, 16)  OutScaling=2^0
  flash : Stateflow chart
  period : Constant  Value=2*pi  OutDataType=fixdt(1, 16)  OutScaling=2^0
  rho0 : Constant  Value=rho0+rand(1)*var  OutDataType=fixdt(1, 16)  OutScaling=2^0
  Out1 : Outport  OutDataType=fixdt(1, 16)  OutScaling=2^0
  wires:
  In20/1 -> Mux/19
  In19/1 -> Mux/18
  In17/1 -> Mux/17
  In16/1 -> Mux/16
  In15/1 -> Mux/15
  In14/1 -> Mux/14
  In13/1 -> Mux/13
  In12/1 -> Mux/12
  In11/1 -> Mux/11
  In10/1 -> Mux/10
  In9/1 -> Mux/9
  In8/1 -> Mux/8
  In7/1 -> Mux/7
  In6/1 -> Mux/6
  In5/1 -> Mux/5
  In4/1 -> Mux/4
  In3/1 -> Mux/3
  In2/1 -> Mux/2
  Threshold/1 -> flash/2(t)
  Math Function/1 -> flash/1(u), Scope2/1
  period/1 -> Math Function/2
  rho0/1 -> Integrator/2
  Sum of Elements/1 -> Gain/1
  Trigonometric Function/1 -> Sum of Elements/1
  Add/1 -> Integrator/1  "drho/dt"
  Gain/1 -> Add/2
  angle speed/1 -> Add/1
  Add1/1 -> Trigonometric Function/1
  Integrator/1 -> Math Function/1, Scope/1, Out1/1, Add1/2  "rho_i"
  Mux/1 -> Add1/1
  In1/1 -> Mux/1

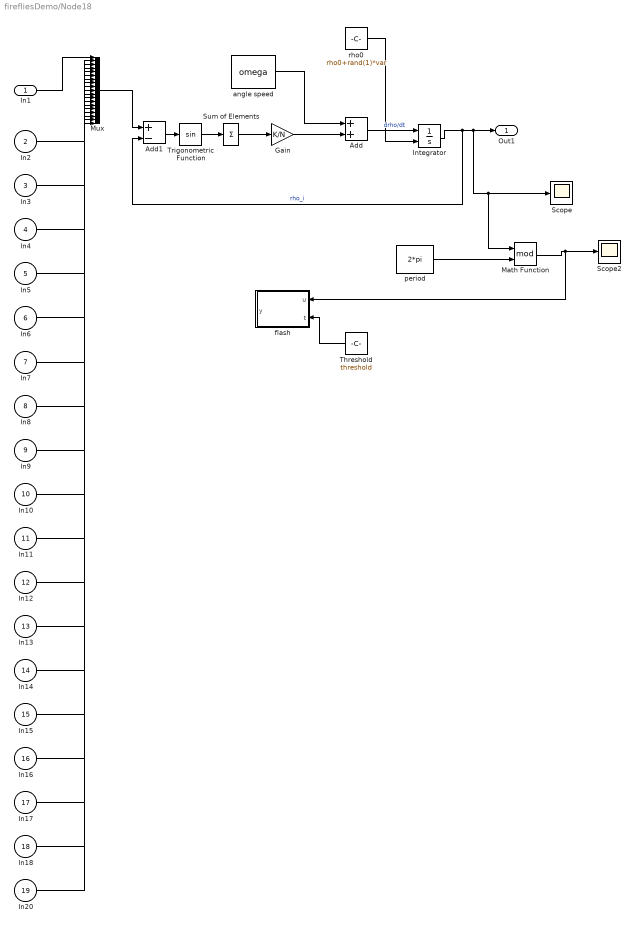
== system firefliesDemo/Node18 ==
  In1 : Inport  OutDataType=fixdt(1, 16)  OutScaling=2^0
  In2 : Inport  Port=2
  In3 : Inport  Port=3
  In4 : Inport  Port=4
  In5 : Inport  Port=5
  In6 : Inport  Port=6
  In7 : Inport  Port=7
  In8 : Inport  Port=8
  In9 : Inport  Port=9
  In10 : Inport  Port=10
  In11 : Inport  Port=11
  In12 : Inport  Port=12
  In13 : Inport  Port=13
  In14 : Inport  Port=14
  In15 : Inport  Port=15
  In16 : Inport  Port=16
  In17 : Inport  Port=17
  In18 : Inport  Port=18
  In20 : Inport  Port=19
  Add : Sum  OutDataType=fixdt(1, 16)  OutScaling=2^-10
  Add1 : Sum  Inputs=+-  OutDataType=fixdt(1, 16)  OutScaling=2^-10
  Gain : Gain  Gain=K/N  ParameterDataType=fixdt(1, 16)  ParameterScaling=2^0  OutDataType=fixdt(1, 16)  OutScaling=2^0
  Integrator : Integrator  InitialConditionSource=external
  Math Function : Math  Operator=mod  OutDataType=fixdt(1, 16)  OutScaling=2^0  SaturateOnIntegerOverflow=on
  Mux : Mux  Inputs=19
  Scope : Scope
  Scope2 : Scope
      settings: SaveName=ScopeData2
  Sum of Elements : Sum  Inputs=+  OutDataType=fixdt(1, 16)  OutScaling=2^-10
  Threshold : Constant  Value=threshold  OutDataType=fixdt(1, 16)  OutScaling=2^0
  Trigonometric Function : Trigonometry
  angle speed : Constant  Value=omega  OutDataType=fixdt(1, 16)  OutScaling=2^0
  flash : Stateflow chart
  period : Constant  Value=2*pi  OutDataType=fixdt(1, 16)  OutScaling=2^0
  rho0 : Constant  Value=rho0+rand(1)*var  OutDataType=fixdt(1, 16)  OutScaling=2^0
  Out1 : Outport  OutDataType=fixdt(1, 16)  OutScaling=2^0
  wires:
  In20/1 -> Mux/19
  In18/1 -> Mux/18
  In17/1 -> Mux/17
  In16/1 -> Mux/16
  In15/1 -> Mux/15
  In14/1 -> Mux/14
  In13/1 -> Mux/13
  In12/1 -> Mux/12
  In11/1 -> Mux/11
  In10/1 -> Mux/10
  In9/1 -> Mux/9
  In8/1 -> Mux/8
  In7/1 -> Mux/7
  In6/1 -> Mux/6
  In5/1 -> Mux/5
  In4/1 -> Mux/4
  In3/1 -> Mux/3
  In2/1 -> Mux/2
  Threshold/1 -> flash/2(t)
  Math Function/1 -> flash/1(u), Scope2/1
  period/1 -> Math Function/2
  rho0/1 -> Integrator/2
  Sum of Elements/1 -> Gain/1
  Trigonometric Function/1 -> Sum of Elements/1
  Add/1 -> Integrator/1  "drho/dt"
  Gain/1 -> Add/2
  angle speed/1 -> Add/1
  Add1/1 -> Trigonometric Function/1
  Integrator/1 -> Math Function/1, Scope/1, Out1/1, Add1/2  "rho_i"
  Mux/1 -> Add1/1
  In1/1 -> Mux/1

== system firefliesDemo/Node19 ==
  In1 : Inport  OutDataType=fixdt(1, 16)  OutScaling=2^0
  In2 : Inport  Port=2
  In3 : Inport  Port=3
  In4 : Inport  Port=4
  In5 : Inport  Port=5
  In6 : Inport  Port=6
  In7 : Inport  Port=7
  In8 : Inport  Port=8
  In9 : Inport  Port=9
  In10 : Inport  Port=10
  In11 : Inport  Port=11
  In12 : Inport  Port=12
  In13 : Inport  Port=13
  In14 : Inport  Port=14
  In15 : Inport  Port=15
  In16 : Inport  Port=16
  In17 : Inport  Port=17
  In18 : Inport  Port=18
  In19 : Inport  Port=19
  Add : Sum  OutDataType=fixdt(1, 16)  OutScaling=2^-10
  Add1 : Sum  Inputs=+-  OutDataType=fixdt(1, 16)  OutScaling=2^-10
  Gain : Gain  Gain=K/N  ParameterDataType=fixdt(1, 16)  ParameterScaling=2^0  OutDataType=fixdt(1, 16)  OutScaling=2^0
  Integrator : Integrator  InitialConditionSource=external
  Math Function : Math  Operator=mod  OutDataType=fixdt(1, 16)  OutScaling=2^0  SaturateOnIntegerOverflow=on
  Mux : Mux  Inputs=19
  Scope : Scope
  Scope2 : Scope
      settings: SaveName=ScopeData2
  Sum of Elements : Sum  Inputs=+  OutDataType=fixdt(1, 16)  OutScaling=2^-10
  Threshold : Constant  Value=threshold  OutDataType=fixdt(1, 16)  OutScaling=2^0
  Trigonometric Function : Trigonometry
  angle speed : Constant  Value=omega  OutDataType=fixdt(1, 16)  OutScaling=2^0
  flash : Stateflow chart
  period : Constant  Value=2*pi  OutDataType=fixdt(1, 16)  OutScaling=2^0
  rho0 : Constant  Value=rho0+rand(1)*var  OutDataType=fixdt(1, 16)  OutScaling=2^0
  Out1 : Outport  OutDataType=fixdt(1, 16)  OutScaling=2^0
  wires:
  In19/1 -> Mux/19
  In18/1 -> Mux/18
  In17/1 -> Mux/17
  In16/1 -> Mux/16
  In15/1 -> Mux/15
  In14/1 -> Mux/14
  In13/1 -> Mux/13
  In12/1 -> Mux/12
  In11/1 -> Mux/11
  In10/1 -> Mux/10
  In9/1 -> Mux/9
  In8/1 -> Mux/8
  In7/1 -> Mux/7
  In6/1 -> Mux/6
  In5/1 -> Mux/5
  In4/1 -> Mux/4
  In3/1 -> Mux/3
  In2/1 -> Mux/2
  Threshold/1 -> flash/2(t)
  Math Function/1 -> flash/1(u), Scope2/1
  period/1 -> Math Function/2
  rho0/1 -> Integrator/2
  Sum of Elements/1 -> Gain/1
  Trigonometric Function/1 -> Sum of Elements/1
  Add/1 -> Integrator/1  "drho/dt"
  Gain/1 -> Add/2
  angle speed/1 -> Add/1
  Add1/1 -> Trigonometric Function/1
  Integrator/1 -> Math Function/1, Scope/1, Out1/1, Add1/2  "rho_i"
  Mux/1 -> Add1/1
  In1/1 -> Mux/1

== system firefliesDemo/Node2 ==
  In1 : Inport  OutDataType=fixdt(1, 16)  OutScaling=2^0
  In2 : Inport  Port=2
  In4 : Inport  Port=3
  In5 : Inport  Port=4
  In6 : Inport  Port=5
  In7 : Inport  Port=6
  In8 : Inport  Port=7
  In9 : Inport  Port=8
  In10 : Inport  Port=9
  In11 : Inport  Port=10
  In12 : Inport  Port=11
  In13 : Inport  Port=12
  In14 : Inport  Port=13
  In15 : Inport  Port=14
  In16 : Inport  Port=15
  In17 : Inport  Port=16
  In18 : Inport  Port=17
  In19 : Inport  Port=18
  In20 : Inport  Port=19
  Add : Sum  OutDataType=fixdt(1, 16)  OutScaling=2^-10
  Add1 : Sum  Inputs=+-  OutDataType=fixdt(1, 16)  OutScaling=2^-10
  Gain : Gain  Gain=K/N  ParameterDataType=fixdt(1, 16)  ParameterScaling=2^0  OutDataType=fixdt(1, 16)  OutScaling=2^0
  Integrator : Integrator  InitialConditionSource=external
  Math Function : Math  Operator=mod  OutDataType=fixdt(1, 16)  OutScaling=2^0  SaturateOnIntegerOverflow=on
  Mux : Mux  Inputs=19
  Scope : Scope
  Scope2 : Scope
      settings: SaveName=ScopeData2
  Sum of Elements : Sum  Inputs=+  OutDataType=fixdt(1, 16)  OutScaling=2^-10
  Threshold : Constant  Value=threshold  OutDataType=fixdt(1, 16)  OutScaling=2^0
  Trigonometric Function : Trigonometry
  angle speed : Constant  Value=omega  OutDataType=fixdt(1, 16)  OutScaling=2^0
  flash : Stateflow chart
  period : Constant  Value=2*pi  OutDataType=fixdt(1, 16)  OutScaling=2^0
  rho0 : Constant  Value=rho0+rand(1)*var  OutDataType=fixdt(1, 16)  OutScaling=2^0
  Out1 : Outport  OutDataType=fixdt(1, 16)  OutScaling=2^0
  wires:
  In20/1 -> Mux/19
  In19/1 -> Mux/18
  In18/1 -> Mux/17
  In17/1 -> Mux/16
  In16/1 -> Mux/15
  In15/1 -> Mux/14
  In14/1 -> Mux/13
  In13/1 -> Mux/12
  In12/1 -> Mux/11
  In11/1 -> Mux/10
  In10/1 -> Mux/9
  In9/1 -> Mux/8
  In8/1 -> Mux/7
  In7/1 -> Mux/6
  In6/1 -> Mux/5
  In5/1 -> Mux/4
  In4/1 -> Mux/3
  In2/1 -> Mux/2
  Threshold/1 -> flash/2(t)
  Math Function/1 -> flash/1(u), Scope2/1
  period/1 -> Math Function/2
  rho0/1 -> Integrator/2
  Sum of Elements/1 -> Gain/1
  Trigonometric Function/1 -> Sum of Elements/1
  Add/1 -> Integrator/1  "drho/dt"
  Gain/1 -> Add/2
  angle speed/1 -> Add/1
  Add1/1 -> Trigonometric Function/1
  Integrator/1 -> Math Function/1, Scope/1, Out1/1, Add1/2  "rho_i"
  Mux/1 -> Add1/1
  In1/1 -> Mux/1

== system firefliesDemo/Node3 ==
  In1 : Inport  OutDataType=fixdt(1, 16)  OutScaling=2^0
  In2 : Inport  Port=2
  In3 : Inport  Port=3
  In5 : Inport  Port=4
  In6 : Inport  Port=5
  In7 : Inport  Port=6
  In8 : Inport  Port=7
  In9 : Inport  Port=8
  In10 : Inport  Port=9
  In11 : Inport  Port=10
  In12 : Inport  Port=11
  In13 : Inport  Port=12
  In14 : Inport  Port=13
  In15 : Inport  Port=14
  In16 : Inport  Port=15
  In17 : Inport  Port=16
  In18 : Inport  Port=17
  In19 : Inport  Port=18
  In20 : Inport  Port=19
  Add : Sum  OutDataType=fixdt(1, 16)  OutScaling=2^-10
  Add1 : Sum  Inputs=+-  OutDataType=fixdt(1, 16)  OutScaling=2^-10
  Gain : Gain  Gain=K/N  ParameterDataType=fixdt(1, 16)  ParameterScaling=2^0  OutDataType=fixdt(1, 16)  OutScaling=2^0
  Integrator : Integrator  InitialConditionSource=external
  Math Function : Math  Operator=mod  OutDataType=fixdt(1, 16)  OutScaling=2^0  SaturateOnIntegerOverflow=on
  Mux : Mux  Inputs=19
  Scope : Scope
  Scope2 : Scope
      settings: SaveName=ScopeData2
  Sum of Elements : Sum  Inputs=+  OutDataType=fixdt(1, 16)  OutScaling=2^-10
  Threshold : Constant  Value=threshold  OutDataType=fixdt(1, 16)  OutScaling=2^0
  Trigonometric Function : Trigonometry
  angle speed : Constant  Value=omega  OutDataType=fixdt(1, 16)  OutScaling=2^0
  flash : Stateflow chart
  period : Constant  Value=2*pi  OutDataType=fixdt(1, 16)  OutScaling=2^0
  rho0 : Constant  Value=rho0+rand(1)*var  OutDataType=fixdt(1, 16)  OutScaling=2^0
  Out1 : Outport  OutDataType=fixdt(1, 16)  OutScaling=2^0
  wires:
  In20/1 -> Mux/19
  In19/1 -> Mux/18
  In18/1 -> Mux/17
  In17/1 -> Mux/16
  In16/1 -> Mux/15
  In15/1 -> Mux/14
  In14/1 -> Mux/13
  In13/1 -> Mux/12
  In12/1 -> Mux/11
  In11/1 -> Mux/10
  In10/1 -> Mux/9
  In9/1 -> Mux/8
  In8/1 -> Mux/7
  In7/1 -> Mux/6
  In6/1 -> Mux/5
  In5/1 -> Mux/4
  In3/1 -> Mux/3
  In2/1 -> Mux/2
  Threshold/1 -> flash/2(t)
  Math Function/1 -> flash/1(u), Scope2/1
  period/1 -> Math Function/2
  rho0/1 -> Integrator/2
  Sum of Elements/1 -> Gain/1
  Trigonometric Function/1 -> Sum of Elements/1
  Add/1 -> Integrator/1  "drho/dt"
  Gain/1 -> Add/2
  angle speed/1 -> Add/1
  Add1/1 -> Trigonometric Function/1
  Integrator/1 -> Math Function/1, Scope/1, Out1/1, Add1/2  "rho_i"
  Mux/1 -> Add1/1
  In1/1 -> Mux/1

== system firefliesDemo/Node4 ==
  In1 : Inport  OutDataType=fixdt(1, 16)  OutScaling=2^0
  In2 : Inport  Port=2
  In3 : Inport  Port=3
  In4 : Inport  Port=4
  In6 : Inport  Port=5
  In7 : Inport  Port=6
  In8 : Inport  Port=7
  In9 : Inport  Port=8
  In10 : Inport  Port=9
  In11 : Inport  Port=10
  In12 : Inport  Port=11
  In13 : Inport  Port=12
  In14 : Inport  Port=13
  In15 : Inport  Port=14
  In16 : Inport  Port=15
  In17 : Inport  Port=16
  In18 : Inport  Port=17
  In19 : Inport  Port=18
  In20 : Inport  Port=19
  Add : Sum  OutDataType=fixdt(1, 16)  OutScaling=2^-10
  Add1 : Sum  Inputs=+-  OutDataType=fixdt(1, 16)  OutScaling=2^-10
  Gain : Gain  Gain=K/N  ParameterDataType=fixdt(1, 16)  ParameterScaling=2^0  OutDataType=fixdt(1, 16)  OutScaling=2^0
  Integrator : Integrator  InitialConditionSource=external
  Math Function : Math  Operator=mod  OutDataType=fixdt(1, 16)  OutScaling=2^0  SaturateOnIntegerOverflow=on
  Mux : Mux  Inputs=19
  Scope : Scope
  Scope2 : Scope
      settings: SaveName=ScopeData2
  Sum of Elements : Sum  Inputs=+  OutDataType=fixdt(1, 16)  OutScaling=2^-10
  Threshold : Constant  Value=threshold  OutDataType=fixdt(1, 16)  OutScaling=2^0
  Trigonometric Function : Trigonometry
  angle speed : Constant  Value=omega  OutDataType=fixdt(1, 16)  OutScaling=2^0
  flash : Stateflow chart
  period : Constant  Value=2*pi  OutDataType=fixdt(1, 16)  OutScaling=2^0
  rho0 : Constant  Value=rho0+rand(1)*var  OutDataType=fixdt(1, 16)  OutScaling=2^0
  Out1 : Outport  OutDataType=fixdt(1, 16)  OutScaling=2^0
  wires:
  In20/1 -> Mux/19
  In19/1 -> Mux/18
  In18/1 -> Mux/17
  In17/1 -> Mux/16
  In16/1 -> Mux/15
  In15/1 -> Mux/14
  In14/1 -> Mux/13
  In13/1 -> Mux/12
  In12/1 -> Mux/11
  In11/1 -> Mux/10
  In10/1 -> Mux/9
  In9/1 -> Mux/8
  In8/1 -> Mux/7
  In7/1 -> Mux/6
  In6/1 -> Mux/5
  In4/1 -> Mux/4
  In3/1 -> Mux/3
  In2/1 -> Mux/2
  Threshold/1 -> flash/2(t)
  Math Function/1 -> flash/1(u), Scope2/1
  period/1 -> Math Function/2
  rho0/1 -> Integrator/2
  Sum of Elements/1 -> Gain/1
  Trigonometric Function/1 -> Sum of Elements/1
  Add/1 -> Integrator/1  "drho/dt"
  Gain/1 -> Add/2
  angle speed/1 -> Add/1
  Add1/1 -> Trigonometric Function/1
  Integrator/1 -> Math Function/1, Scope/1, Out1/1, Add1/2  "rho_i"
  Mux/1 -> Add1/1
  In1/1 -> Mux/1

== system firefliesDemo/Node5 ==
  In1 : Inport  OutDataType=fixdt(1, 16)  OutScaling=2^0
  In2 : Inport  Port=2
  In3 : Inport  Port=3
  In4 : Inport  Port=4
  In5 : Inport  Port=5
  In7 : Inport  Port=6
  In8 : Inport  Port=7
  In9 : Inport  Port=8
  In10 : Inport  Port=9
  In11 : Inport  Port=10
  In12 : Inport  Port=11
  In13 : Inport  Port=12
  In14 : Inport  Port=13
  In15 : Inport  Port=14
  In16 : Inport  Port=15
  In17 : Inport  Port=16
  In18 : Inport  Port=17
  In19 : Inport  Port=18
  In20 : Inport  Port=19
  Add : Sum  OutDataType=fixdt(1, 16)  OutScaling=2^-10
  Add1 : Sum  Inputs=+-  OutDataType=fixdt(1, 16)  OutScaling=2^-10
  Gain : Gain  Gain=K/N  ParameterDataType=fixdt(1, 16)  ParameterScaling=2^0  OutDataType=fixdt(1, 16)  OutScaling=2^0
  Integrator : Integrator  InitialConditionSource=external
  Math Function : Math  Operator=mod  OutDataType=fixdt(1, 16)  OutScaling=2^0  SaturateOnIntegerOverflow=on
  Mux : Mux  Inputs=19
  Scope : Scope
  Scope2 : Scope
      settings: SaveName=ScopeData2
  Sum of Elements : Sum  Inputs=+  OutDataType=fixdt(1, 16)  OutScaling=2^-10
  Threshold : Constant  Value=threshold  OutDataType=fixdt(1, 16)  OutScaling=2^0
  Trigonometric Function : Trigonometry
  angle speed : Constant  Value=omega  OutDataType=fixdt(1, 16)  OutScaling=2^0
  flash : Stateflow chart
  period : Constant  Value=2*pi  OutDataType=fixdt(1, 16)  OutScaling=2^0
  rho0 : Constant  Value=rho0+rand(1)*var  OutDataType=fixdt(1, 16)  OutScaling=2^0
  Out1 : Outport  OutDataType=fixdt(1, 16)  OutScaling=2^0
  wires:
  In20/1 -> Mux/19
  In19/1 -> Mux/18
  In18/1 -> Mux/17
  In17/1 -> Mux/16
  In16/1 -> Mux/15
  In15/1 -> Mux/14
  In14/1 -> Mux/13
  In13/1 -> Mux/12
  In12/1 -> Mux/11
  In11/1 -> Mux/10
  In10/1 -> Mux/9
  In9/1 -> Mux/8
  In8/1 -> Mux/7
  In7/1 -> Mux/6
  In5/1 -> Mux/5
  In4/1 -> Mux/4
  In3/1 -> Mux/3
  In2/1 -> Mux/2
  Threshold/1 -> flash/2(t)
  Math Function/1 -> flash/1(u), Scope2/1
  period/1 -> Math Function/2
  rho0/1 -> Integrator/2
  Sum of Elements/1 -> Gain/1
  Trigonometric Function/1 -> Sum of Elements/1
  Add/1 -> Integrator/1  "drho/dt"
  Gain/1 -> Add/2
  angle speed/1 -> Add/1
  Add1/1 -> Trigonometric Function/1
  Integrator/1 -> Math Function/1, Scope/1, Out1/1, Add1/2  "rho_i"
  Mux/1 -> Add1/1
  In1/1 -> Mux/1

== system firefliesDemo/Node6 ==
  In1 : Inport  OutDataType=fixdt(1, 16)  OutScaling=2^0
  In2 : Inport  Port=2
  In3 : Inport  Port=3
  In4 : Inport  Port=4
  In5 : Inport  Port=5
  In6 : Inport  Port=6
  In8 : Inport  Port=7
  In9 : Inport  Port=8
  In10 : Inport  Port=9
  In11 : Inport  Port=10
  In12 : Inport  Port=11
  In13 : Inport  Port=12
  In14 : Inport  Port=13
  In15 : Inport  Port=14
  In16 : Inport  Port=15
  In17 : Inport  Port=16
  In18 : Inport  Port=17
  In19 : Inport  Port=18
  In20 : Inport  Port=19
  Add : Sum  OutDataType=fixdt(1, 16)  OutScaling=2^-10
  Add1 : Sum  Inputs=+-  OutDataType=fixdt(1, 16)  OutScaling=2^-10
  Gain : Gain  Gain=K/N  ParameterDataType=fixdt(1, 16)  ParameterScaling=2^0  OutDataType=fixdt(1, 16)  OutScaling=2^0
  Integrator : Integrator  InitialConditionSource=external
  Math Function : Math  Operator=mod  OutDataType=fixdt(1, 16)  OutScaling=2^0  SaturateOnIntegerOverflow=on
  Mux : Mux  Inputs=19
  Scope : Scope
  Scope2 : Scope
      settings: SaveName=ScopeData2
  Sum of Elements : Sum  Inputs=+  OutDataType=fixdt(1, 16)  OutScaling=2^-10
  Threshold : Constant  Value=threshold  OutDataType=fixdt(1, 16)  OutScaling=2^0
  Trigonometric Function : Trigonometry
  angle speed : Constant  Value=omega  OutDataType=fixdt(1, 16)  OutScaling=2^0
  flash : Stateflow chart
  period : Constant  Value=2*pi  OutDataType=fixdt(1, 16)  OutScaling=2^0
  rho0 : Constant  Value=rho0+rand(1)*var  OutDataType=fixdt(1, 16)  OutScaling=2^0
  Out1 : Outport  OutDataType=fixdt(1, 16)  OutScaling=2^0
  wires:
  In20/1 -> Mux/19
  In19/1 -> Mux/18
  In18/1 -> Mux/17
  In17/1 -> Mux/16
  In16/1 -> Mux/15
  In15/1 -> Mux/14
  In14/1 -> Mux/13
  In13/1 -> Mux/12
  In12/1 -> Mux/11
  In11/1 -> Mux/10
  In10/1 -> Mux/9
  In9/1 -> Mux/8
  In8/1 -> Mux/7
  In6/1 -> Mux/6
  In5/1 -> Mux/5
  In4/1 -> Mux/4
  In3/1 -> Mux/3
  In2/1 -> Mux/2
  Threshold/1 -> flash/2(t)
  Math Function/1 -> flash/1(u), Scope2/1
  period/1 -> Math Function/2
  rho0/1 -> Integrator/2
  Sum of Elements/1 -> Gain/1
  Trigonometric Function/1 -> Sum of Elements/1
  Add/1 -> Integrator/1  "drho/dt"
  Gain/1 -> Add/2
  angle speed/1 -> Add/1
  Add1/1 -> Trigonometric Function/1
  Integrator/1 -> Math Function/1, Scope/1, Out1/1, Add1/2  "rho_i"
  Mux/1 -> Add1/1
  In1/1 -> Mux/1

== system firefliesDemo/Node7 ==
  In1 : Inport  OutDataType=fixdt(1, 16)  OutScaling=2^0
  In2 : Inport  Port=2
  In3 : Inport  Port=3
  In4 : Inport  Port=4
  In5 : Inport  Port=5
  In6 : Inport  Port=6
  In7 : Inport  Port=7
  In9 : Inport  Port=8
  In10 : Inport  Port=9
  In11 : Inport  Port=10
  In12 : Inport  Port=11
  In13 : Inport  Port=12
  In14 : Inport  Port=13
  In15 : Inport  Port=14
  In16 : Inport  Port=15
  In17 : Inport  Port=16
  In18 : Inport  Port=17
  In19 : Inport  Port=18
  In20 : Inport  Port=19
  Add : Sum  OutDataType=fixdt(1, 16)  OutScaling=2^-10
  Add1 : Sum  Inputs=+-  OutDataType=fixdt(1, 16)  OutScaling=2^-10
  Gain : Gain  Gain=K/N  ParameterDataType=fixdt(1, 16)  ParameterScaling=2^0  OutDataType=fixdt(1, 16)  OutScaling=2^0
  Integrator : Integrator  InitialConditionSource=external
  Math Function : Math  Operator=mod  OutDataType=fixdt(1, 16)  OutScaling=2^0  SaturateOnIntegerOverflow=on
  Mux : Mux  Inputs=19
  Scope : Scope
  Scope2 : Scope
      settings: SaveName=ScopeData2
  Sum of Elements : Sum  Inputs=+  OutDataType=fixdt(1, 16)  OutScaling=2^-10
  Threshold : Constant  Value=threshold  OutDataType=fixdt(1, 16)  OutScaling=2^0
  Trigonometric Function : Trigonometry
  angle speed : Constant  Value=omega  OutDataType=fixdt(1, 16)  OutScaling=2^0
  flash : Stateflow chart
  period : Constant  Value=2*pi  OutDataType=fixdt(1, 16)  OutScaling=2^0
  rho0 : Constant  Value=rho0+rand(1)*var  OutDataType=fixdt(1, 16)  OutScaling=2^0
  Out1 : Outport  OutDataType=fixdt(1, 16)  OutScaling=2^0
  wires:
  In20/1 -> Mux/19
  In19/1 -> Mux/18
  In18/1 -> Mux/17
  In17/1 -> Mux/16
  In16/1 -> Mux/15
  In15/1 -> Mux/14
  In14/1 -> Mux/13
  In13/1 -> Mux/12
  In12/1 -> Mux/11
  In11/1 -> Mux/10
  In10/1 -> Mux/9
  In9/1 -> Mux/8
  In7/1 -> Mux/7
  In6/1 -> Mux/6
  In5/1 -> Mux/5
  In4/1 -> Mux/4
  In3/1 -> Mux/3
  In2/1 -> Mux/2
  Threshold/1 -> flash/2(t)
  Math Function/1 -> flash/1(u), Scope2/1
  period/1 -> Math Function/2
  rho0/1 -> Integrator/2
  Sum of Elements/1 -> Gain/1
  Trigonometric Function/1 -> Sum of Elements/1
  Add/1 -> Integrator/1  "drho/dt"
  Gain/1 -> Add/2
  angle speed/1 -> Add/1
  Add1/1 -> Trigonometric Function/1
  Integrator/1 -> Math Function/1, Scope/1, Out1/1, Add1/2  "rho_i"
  Mux/1 -> Add1/1
  In1/1 -> Mux/1
